simulink model "Modelo_benchmark"  (R2023a)
settings: Solver=VariableStepAuto  StartTime=0.0  StopTime=6250  RelTol=1e-3
values from neighbouring files (symbols this model uses):
  A = 0.0012    [control_temperatura.mat]    (also in var.m)
  C1_Q1 = 64.8931891795    [control_temperatura.mat]    (also in var.m = k3*Tau2)
  C1_Q2 = 0.0892445260493    [control_temperatura.mat]    (also in var.m = k1*k6)
  C2_Q1 = 0.558623321055    [control_temperatura.mat]    (also in var.m = k3)
  C_ff = GQ2T1cr/GQ1T1cr    [var.m]
  cp = 500    [control_temperatura.mat]    (also in var.m)
  e = zeros(1,iteraciones+ini)    [Codigo_discreto_ap.m]    (also in control_temperatura.mat = 0.9; var.m = 0.9)
  GQ1T1cr = tf(kcr1, [Taucr1 1])    [var.m]
  Hf1 = 0.01    [control_temperatura.mat]    (also in var.m)
  Hf2 = 0.004    [control_temperatura.mat]    (also in var.m)
  K_ap = 7.31538861094    [control_temperatura.mat]    (also in var.m = (2*delta*Taucr1*wn-1)/kcr1)
  K_cp = 1.15885597738    [control_temperatura.mat]    (also in var.m)
  m = 0.004    [control_temperatura.mat]    (also in var.m)
  P1_Q1 = 12978.6378359    [control_temperatura.mat]    (also in var.m = Tau1*Tau2)
  P1_Q2 = 12978.6378359    [control_temperatura.mat]    (also in var.m = Tau1*Tau2)
  P2_Q1 = 227.890937142    [control_temperatura.mat]    (also in var.m = Tau2+Tau1)
  P2_Q2 = 227.890937142    [control_temperatura.mat]    (also in var.m = Tau2+Tau1)
  P3_Q1 = 0.840856230771    [control_temperatura.mat]    (also in var.m = 1- k1*k4)
  P3_Q2 = 0.840856230771    [control_temperatura.mat]    (also in var.m = 1- k1*k4)
  T1i = 299.55    [control_temperatura.mat]    (also in var.m)
  T1o = 309.62355074    [control_temperatura.mat]    (also in var.m = x(1))
  T2i = 299.55    [control_temperatura.mat]    (also in var.m)
  TA = 299.55    [control_temperatura.mat]    (also in var.m)
  th = 5.67e-08    [control_temperatura.mat]    (also in var.m)
  Ti_ap = 23.6710802631    [control_temperatura.mat]    (also in var.m = (K_ap*kcr1)/(Taucr1*wn^2))
  Ti_cp = 165    [control_temperatura.mat]    (also in var.m)
  Tk = 273.15    [control_temperatura.mat]    (also in var.m)
  Tt_ap = 4.8652934406    [control_temperatura.mat]    (also in var.m = sqrt(Ti_ap))
  Tt_cp = 12.8452325787    [control_temperatura.mat]    (also in var.m = sqrt(Ti_cp))
  U = 1.4    [control_temperatura.mat]    (also in var.m)
undefined symbols (not defined in the file or in its folder): PID_Matlab
libraries: slpidlib x8, simulink_extras x6, simulink x4
(part 1 of 2)
settings Model: PacingRate=10  Creator=User  LastModifiedBy=User

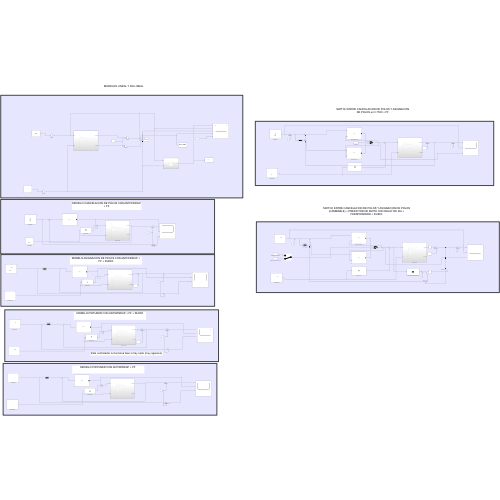
[thumbnail: Simulink's stored preview of the top-level diagram]
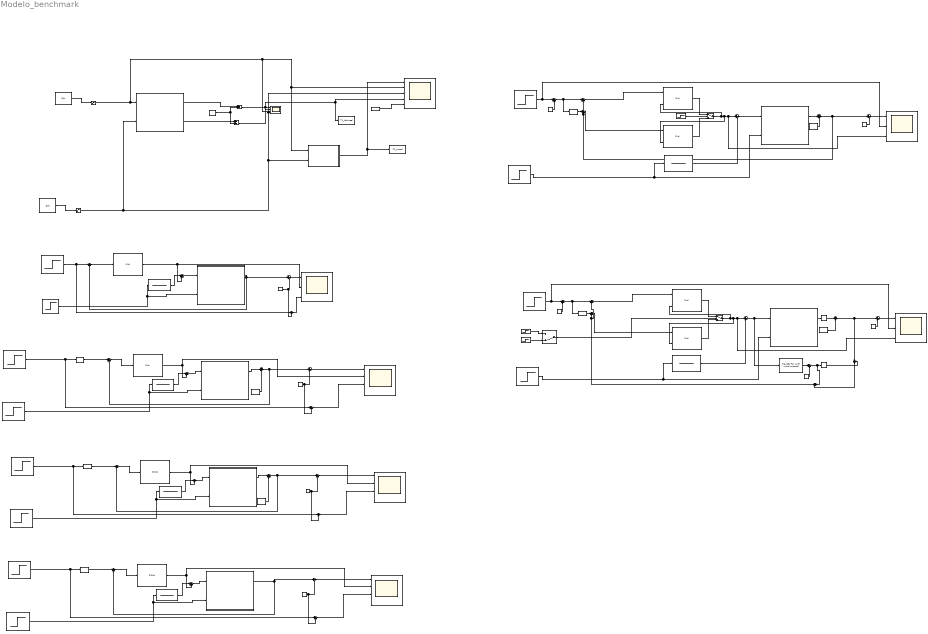
== system Modelo_benchmark ==
  note: SWITCH ENTRE CANCELACION DE POLOS Y ASIGNACION DE POLOS en t=1500 + FF
  note: MODELOS LINEAL Y NO LINEAL
  note: MODELO CANCELACION DE POLOS CON ANTIWINDUP + FF
  note: MODELO ASIGNACION DE POLOS CON ANTIWINDUP + FF + RUIDO
  note: SWITCH ENTRE CANCELACION DE POLOS Y ASIGNACION DE POLOS (CAMBIABLE) + PREDICTOR DE SMITH CON DELAY DE 40s + FEEDFORWARD + RUIDO
  note: MODELO PIDTUNER CON ANTIWINDUP + FF + RUIDO
  note: MODELO PIDTUNER CON ANTIWINDUP + FF
  note: Este controlador no funciona bien si hay ruido (muy agresivo)
  ASIGNACION POLOS : slpidlib/PID Controller  Controller=PI  Form=Parallel  TimeDomain=Continuous-time  UseExternalTs=off  SampleTime=-1  IntegratorMethod=Forward Euler  FilterMethod=Forward Euler  ControllerParametersSource=internal  P=K_ap  I=1/Ti_ap  UseKiTs=off  D=2  N=100  UseFilter=on  TunerSelectOption=Transfer Function Based (PID Tuner App)  InitialConditionSource=internal  InitialConditionForIntegrator=0  InitialConditionForFilter=0  DifferentiatorICPrevScaledInput=0  ExternalReset=none  TrackingMode=on  Kt=1/Tt_ap  LimitOutput=on  SatLimitsSource=internal  UpperSaturationLimit=100  LowerSaturationLimit=0  LinearizeAsGain=on  AntiWindupMode=back-calculation  Kb=1/Tt_ap  LimitIntegrator=off  UpperIntegratorSaturationLimit=inf  LowerIntegratorSaturationLimit=-inf  POutMin=[]  POutMax=[]  IOutMin=[]  IOutMax=[]  DOutMin=[]  DOutMax=[]  NOutMin=[]  NOutMax=[]  SumOutMin=[]  SumOutMax=[]  SaturationOutMin=[]  SaturationOutMax=[]  PParamMin=[]  PParamMax=[]  IParamMin=[]  IParamMax=[]  DParamMin=[]  DParamMax=[]  NParamMin=[]  NParamMax=[]  KbParamMin=[]  KbParamMax=[]  KtParamMin=[]  KtParamMax=[]  KbOutMin=[]  KbOutMax=[]  KtOutMin=[]  KtOutMax=[]  IntegratorOutMin=[]  IntegratorOutMax=[]  FilterOutMin=[]  FilterOutMax=[]  SumI1OutMin=[]  SumI1OutMax=[]  SumI2OutMin=[]  SumI2OutMax=[]  SumI3OutMin=[]  SumI3OutMax=[]  SumI4OutMin=[]  SumI4OutMax=[]  SumDOutMin=[]  SumDOutMax=[]  DifferentiatorOutMin=[]  DifferentiatorOutMax=[]  FilterDiffOutCoefMin=[]  FilterDiffOutCoefMax=[]  ReciprocalOutMin=[]  ReciprocalOutMax=[]  SumDenOutMin=[]  SumDenOutMax=[]  SumNumOutMin=[]  SumNumOutMax=[]  DivideOutMin=[]  DivideOutMax=[]  UdiffTsProdOutMin=[]  UdiffTsProdOutMax=[]  NTsProdOutMin=[]  NTsProdOutMax=[]  UintegralTsProdOutMin=[]  UintegralTsProdOutMax=[]  UngainTsProdOutMin=[]  UngainTsProdOutMax=[]  ClampingZeroOutDataTypeStr=Inherit: Inherit via back propagation  ClampingZeroOutMin=[]  ClampingZeroOutMax=[]  FilterDenConstantOutDataTypeStr=Inherit: Inherit via back propagation  FilterDenConstantOutMin=[]  FilterDenConstantOutMax=[]  PCopyOutDataTypeStr=Inherit: Inherit via back propagation  PCopyOutMin=[]  PCopyOutMax=[]  NCopyOutDataTypeStr=Inherit: Inherit via back propagation  NCopyOutMin=[]  NCopyOutMax=[]  IntegratorContinuousStateAttributes=''  IntegratorStateMustResolveToSignalObject=off  IntegratorRTWStateStorageClass=Auto  FilterContinuousStateAttributes=''  FilterStateMustResolveToSignalObject=off  FilterRTWStateStorageClass=Auto  ParallelPVariant=InternalParameters  IdealPVariant=Disabled  IVariant=InternalParameters  DVariant=Disabled  IntegratorVariant=Continuous  SatVariant=Enabled  AWVariant=BackCalculation  PCopyVariant=Disabled  TRVariant=Enabled  FdbkBlocksVariant=Forward  IdealPFdbkVariant=Disabled  SatFdbkVariant=Disabled  DerivativeFilterVariant=Disabled  NVariant=Disabled  NCopyVariant=Disabled_SignalSpec  FilterICVariant=Disabled  IntegratorICVariant=InternalICs  ExternalResetVariant=Disabled  TRSumVariant=TrackingMode  SumFdbkVariant=Disabled  SumVariant=Sum_PI  TsampFilterVariant=InternalTs  TsampNgainVariant=Passthrough  TsampIntegralVariant=Disabled_SignalSpec  ExternalSaturationOutDataTypeStr=Inherit: Same as second input
  ASIGNACION POLOS1 : slpidlib/PID Controller  Controller=PI  Form=Parallel  TimeDomain=Continuous-time  UseExternalTs=off  SampleTime=-1  IntegratorMethod=Forward Euler  FilterMethod=Forward Euler  ControllerParametersSource=internal  P=K_ap  I=1/Ti_ap  UseKiTs=off  D=2  N=100  UseFilter=on  TunerSelectOption=Transfer Function Based (PID Tuner App)  InitialConditionSource=internal  InitialConditionForIntegrator=0  InitialConditionForFilter=0  DifferentiatorICPrevScaledInput=0  ExternalReset=none  TrackingMode=on  Kt=1/Tt_ap  LimitOutput=on  SatLimitsSource=internal  UpperSaturationLimit=100  LowerSaturationLimit=0  LinearizeAsGain=on  AntiWindupMode=back-calculation  Kb=1/Tt_ap  LimitIntegrator=off  UpperIntegratorSaturationLimit=inf  LowerIntegratorSaturationLimit=-inf  POutMin=[]  POutMax=[]  IOutMin=[]  IOutMax=[]  DOutMin=[]  DOutMax=[]  NOutMin=[]  NOutMax=[]  SumOutMin=[]  SumOutMax=[]  SaturationOutMin=[]  SaturationOutMax=[]  PParamMin=[]  PParamMax=[]  IParamMin=[]  IParamMax=[]  DParamMin=[]  DParamMax=[]  NParamMin=[]  NParamMax=[]  KbParamMin=[]  KbParamMax=[]  KtParamMin=[]  KtParamMax=[]  KbOutMin=[]  KbOutMax=[]  KtOutMin=[]  KtOutMax=[]  IntegratorOutMin=[]  IntegratorOutMax=[]  FilterOutMin=[]  FilterOutMax=[]  SumI1OutMin=[]  SumI1OutMax=[]  SumI2OutMin=[]  SumI2OutMax=[]  SumI3OutMin=[]  SumI3OutMax=[]  SumI4OutMin=[]  SumI4OutMax=[]  SumDOutMin=[]  SumDOutMax=[]  DifferentiatorOutMin=[]  DifferentiatorOutMax=[]  FilterDiffOutCoefMin=[]  FilterDiffOutCoefMax=[]  ReciprocalOutMin=[]  ReciprocalOutMax=[]  SumDenOutMin=[]  SumDenOutMax=[]  SumNumOutMin=[]  SumNumOutMax=[]  DivideOutMin=[]  DivideOutMax=[]  UdiffTsProdOutMin=[]  UdiffTsProdOutMax=[]  NTsProdOutMin=[]  NTsProdOutMax=[]  UintegralTsProdOutMin=[]  UintegralTsProdOutMax=[]  UngainTsProdOutMin=[]  UngainTsProdOutMax=[]  ClampingZeroOutDataTypeStr=Inherit: Inherit via back propagation  ClampingZeroOutMin=[]  ClampingZeroOutMax=[]  FilterDenConstantOutDataTypeStr=Inherit: Inherit via back propagation  FilterDenConstantOutMin=[]  FilterDenConstantOutMax=[]  PCopyOutDataTypeStr=Inherit: Inherit via back propagation  PCopyOutMin=[]  PCopyOutMax=[]  NCopyOutDataTypeStr=Inherit: Inherit via back propagation  NCopyOutMin=[]  NCopyOutMax=[]  IntegratorContinuousStateAttributes=''  IntegratorStateMustResolveToSignalObject=off  IntegratorRTWStateStorageClass=Auto  FilterContinuousStateAttributes=''  FilterStateMustResolveToSignalObject=off  FilterRTWStateStorageClass=Auto  ParallelPVariant=InternalParameters  IdealPVariant=Disabled  IVariant=InternalParameters  DVariant=Disabled  IntegratorVariant=Continuous  SatVariant=Enabled  AWVariant=BackCalculation  PCopyVariant=Disabled  TRVariant=Enabled  FdbkBlocksVariant=Forward  IdealPFdbkVariant=Disabled  SatFdbkVariant=Disabled  DerivativeFilterVariant=Disabled  NVariant=Disabled  NCopyVariant=Disabled_SignalSpec  FilterICVariant=Disabled  IntegratorICVariant=InternalICs  ExternalResetVariant=Disabled  TRSumVariant=TrackingMode  SumFdbkVariant=Disabled  SumVariant=Sum_PI  TsampFilterVariant=InternalTs  TsampNgainVariant=Passthrough  TsampIntegralVariant=Disabled_SignalSpec  ExternalSaturationOutDataTypeStr=Inherit: Same as second input
  Band-Limited White Noise : simulink/Sources/Band-Limited White Noise  Cov=[0.2]  Ts=15  seed=[23341]
  Band-Limited White Noise1 : simulink/Sources/Band-Limited White Noise  Cov=[0.2]  Ts=10  seed=[23341]
  Band-Limited White Noise2 : simulink/Sources/Band-Limited White Noise  Cov=[0.2]  Ts=10  seed=[23341]
  Band-Limited White Noise3 : simulink/Sources/Band-Limited White Noise  Cov=[0.2]  Ts=15  seed=[23341]
  CANCELACION POLOS : slpidlib/PID Controller  Controller=PI  Form=Parallel  TimeDomain=Continuous-time  UseExternalTs=off  SampleTime=-1  IntegratorMethod=Forward Euler  FilterMethod=Forward Euler  ControllerParametersSource=internal  P=K_cp  I=1/Ti_cp  UseKiTs=off  D=2  N=100  UseFilter=on  TunerSelectOption=Transfer Function Based (PID Tuner App)  InitialConditionSource=internal  InitialConditionForIntegrator=0  InitialConditionForFilter=0  DifferentiatorICPrevScaledInput=0  ExternalReset=none  TrackingMode=on  Kt=1/Tt_cp  LimitOutput=on  SatLimitsSource=internal  UpperSaturationLimit=100  LowerSaturationLimit=0  LinearizeAsGain=on  AntiWindupMode=back-calculation  Kb=1/Tt_cp  LimitIntegrator=off  UpperIntegratorSaturationLimit=inf  LowerIntegratorSaturationLimit=-inf  POutMin=[]  POutMax=[]  IOutMin=[]  IOutMax=[]  DOutMin=[]  DOutMax=[]  NOutMin=[]  NOutMax=[]  SumOutMin=[]  SumOutMax=[]  SaturationOutMin=[]  SaturationOutMax=[]  PParamMin=[]  PParamMax=[]  IParamMin=[]  IParamMax=[]  DParamMin=[]  DParamMax=[]  NParamMin=[]  NParamMax=[]  KbParamMin=[]  KbParamMax=[]  KtParamMin=[]  KtParamMax=[]  KbOutMin=[]  KbOutMax=[]  KtOutMin=[]  KtOutMax=[]  IntegratorOutMin=[]  IntegratorOutMax=[]  FilterOutMin=[]  FilterOutMax=[]  SumI1OutMin=[]  SumI1OutMax=[]  SumI2OutMin=[]  SumI2OutMax=[]  SumI3OutMin=[]  SumI3OutMax=[]  SumI4OutMin=[]  SumI4OutMax=[]  SumDOutMin=[]  SumDOutMax=[]  DifferentiatorOutMin=[]  DifferentiatorOutMax=[]  FilterDiffOutCoefMin=[]  FilterDiffOutCoefMax=[]  ReciprocalOutMin=[]  ReciprocalOutMax=[]  SumDenOutMin=[]  SumDenOutMax=[]  SumNumOutMin=[]  SumNumOutMax=[]  DivideOutMin=[]  DivideOutMax=[]  UdiffTsProdOutMin=[]  UdiffTsProdOutMax=[]  NTsProdOutMin=[]  NTsProdOutMax=[]  UintegralTsProdOutMin=[]  UintegralTsProdOutMax=[]  UngainTsProdOutMin=[]  UngainTsProdOutMax=[]  ClampingZeroOutDataTypeStr=Inherit: Inherit via back propagation  ClampingZeroOutMin=[]  ClampingZeroOutMax=[]  FilterDenConstantOutDataTypeStr=Inherit: Inherit via back propagation  FilterDenConstantOutMin=[]  FilterDenConstantOutMax=[]  PCopyOutDataTypeStr=Inherit: Inherit via back propagation  PCopyOutMin=[]  PCopyOutMax=[]  NCopyOutDataTypeStr=Inherit: Inherit via back propagation  NCopyOutMin=[]  NCopyOutMax=[]  IntegratorContinuousStateAttributes=''  IntegratorStateMustResolveToSignalObject=off  IntegratorRTWStateStorageClass=Auto  FilterContinuousStateAttributes=''  FilterStateMustResolveToSignalObject=off  FilterRTWStateStorageClass=Auto  ParallelPVariant=InternalParameters  IdealPVariant=Disabled  IVariant=InternalParameters  DVariant=Disabled  IntegratorVariant=Continuous  SatVariant=Enabled  AWVariant=BackCalculation  PCopyVariant=Disabled  TRVariant=Enabled  FdbkBlocksVariant=Forward  IdealPFdbkVariant=Disabled  SatFdbkVariant=Disabled  DerivativeFilterVariant=Disabled  NVariant=Disabled  NCopyVariant=Disabled_SignalSpec  FilterICVariant=Disabled  IntegratorICVariant=InternalICs  ExternalResetVariant=Disabled  TRSumVariant=TrackingMode  SumFdbkVariant=Disabled  SumVariant=Sum_PI  TsampFilterVariant=InternalTs  TsampNgainVariant=Passthrough  TsampIntegralVariant=Disabled_SignalSpec  ExternalSaturationOutDataTypeStr=Inherit: Same as second input
  CANCELACION POLOS1 : slpidlib/PID Controller  Controller=PI  Form=Parallel  TimeDomain=Continuous-time  UseExternalTs=off  SampleTime=-1  IntegratorMethod=Forward Euler  FilterMethod=Forward Euler  ControllerParametersSource=internal  P=K_cp  I=1/Ti_cp  UseKiTs=off  D=2  N=100  UseFilter=on  TunerSelectOption=Transfer Function Based (PID Tuner App)  InitialConditionSource=internal  InitialConditionForIntegrator=0  InitialConditionForFilter=0  DifferentiatorICPrevScaledInput=0  ExternalReset=none  TrackingMode=on  Kt=1/Tt_cp  LimitOutput=on  SatLimitsSource=internal  UpperSaturationLimit=100  LowerSaturationLimit=0  LinearizeAsGain=on  AntiWindupMode=back-calculation  Kb=1/Tt_cp  LimitIntegrator=off  UpperIntegratorSaturationLimit=inf  LowerIntegratorSaturationLimit=-inf  POutMin=[]  POutMax=[]  IOutMin=[]  IOutMax=[]  DOutMin=[]  DOutMax=[]  NOutMin=[]  NOutMax=[]  SumOutMin=[]  SumOutMax=[]  SaturationOutMin=[]  SaturationOutMax=[]  PParamMin=[]  PParamMax=[]  IParamMin=[]  IParamMax=[]  DParamMin=[]  DParamMax=[]  NParamMin=[]  NParamMax=[]  KbParamMin=[]  KbParamMax=[]  KtParamMin=[]  KtParamMax=[]  KbOutMin=[]  KbOutMax=[]  KtOutMin=[]  KtOutMax=[]  IntegratorOutMin=[]  IntegratorOutMax=[]  FilterOutMin=[]  FilterOutMax=[]  SumI1OutMin=[]  SumI1OutMax=[]  SumI2OutMin=[]  SumI2OutMax=[]  SumI3OutMin=[]  SumI3OutMax=[]  SumI4OutMin=[]  SumI4OutMax=[]  SumDOutMin=[]  SumDOutMax=[]  DifferentiatorOutMin=[]  DifferentiatorOutMax=[]  FilterDiffOutCoefMin=[]  FilterDiffOutCoefMax=[]  ReciprocalOutMin=[]  ReciprocalOutMax=[]  SumDenOutMin=[]  SumDenOutMax=[]  SumNumOutMin=[]  SumNumOutMax=[]  DivideOutMin=[]  DivideOutMax=[]  UdiffTsProdOutMin=[]  UdiffTsProdOutMax=[]  NTsProdOutMin=[]  NTsProdOutMax=[]  UintegralTsProdOutMin=[]  UintegralTsProdOutMax=[]  UngainTsProdOutMin=[]  UngainTsProdOutMax=[]  ClampingZeroOutDataTypeStr=Inherit: Inherit via back propagation  ClampingZeroOutMin=[]  ClampingZeroOutMax=[]  FilterDenConstantOutDataTypeStr=Inherit: Inherit via back propagation  FilterDenConstantOutMin=[]  FilterDenConstantOutMax=[]  PCopyOutDataTypeStr=Inherit: Inherit via back propagation  PCopyOutMin=[]  PCopyOutMax=[]  NCopyOutDataTypeStr=Inherit: Inherit via back propagation  NCopyOutMin=[]  NCopyOutMax=[]  IntegratorContinuousStateAttributes=''  IntegratorStateMustResolveToSignalObject=off  IntegratorRTWStateStorageClass=Auto  FilterContinuousStateAttributes=''  FilterStateMustResolveToSignalObject=off  FilterRTWStateStorageClass=Auto  ParallelPVariant=InternalParameters  IdealPVariant=Disabled  IVariant=InternalParameters  DVariant=Disabled  IntegratorVariant=Continuous  SatVariant=Enabled  AWVariant=BackCalculation  PCopyVariant=Disabled  TRVariant=Enabled  FdbkBlocksVariant=Forward  IdealPFdbkVariant=Disabled  SatFdbkVariant=Disabled  DerivativeFilterVariant=Disabled  NVariant=Disabled  NCopyVariant=Disabled_SignalSpec  FilterICVariant=Disabled  IntegratorICVariant=InternalICs  ExternalResetVariant=Disabled  TRSumVariant=TrackingMode  SumFdbkVariant=Disabled  SumVariant=Sum_PI  TsampFilterVariant=InternalTs  TsampNgainVariant=Passthrough  TsampIntegralVariant=Disabled_SignalSpec  ExternalSaturationOutDataTypeStr=Inherit: Same as second input
  Constant{1..6,8..9,14} (9 alike) : Constant  Value=Tk
  Constant7 : Constant  Value=T1i
  Controlador FF{,1..5} (6 alike) : TransferFcn  Numerator=C_ff.Numerator{:}  Denominator=C_ff.Denominator{:}
  From Workspace : FromWorkspace  VariableName=Q1t  SampleTime=0.5
  From Workspace1 : FromWorkspace  VariableName=Q2t  SampleTime=0.5
  From Workspace2 : FromWorkspace  VariableName=T1t
  "MODELO SISTEMA CURVA REACCION " : simulink_extras/Additional Linear/Transfer Fcn (with initial outputs)  N=GQ1T1cr.Numerator{:}  D=GQ1T1cr.Denominator{:}  Y0=0  U0=0
  Manual Switch : ManualSwitch  CurrentSetting=0
  Modelo_ Nolineal : Subsystem
  Modelo_ Nolineal1 : Subsystem
  Modelo_ Nolineal2 : Subsystem
  Modelo_ Nolineal3 : Subsystem
  Modelo_ Nolineal4 : Subsystem
  Modelo_ Nolineal5 : Subsystem
  Modelo_ Nolineal6 : Subsystem
  PERTURBACION : Step  Time=4500  After=15  SampleTime=0
  PERTURBACION{1..5} (5 alike) : Step  Time=4500  After=100  SampleTime=0
  PID Controller : slpidlib/PID Controller  Controller=PI  Form=Parallel  TimeDomain=Continuous-time  UseExternalTs=off  SampleTime=-1  IntegratorMethod=Forward Euler  FilterMethod=Forward Euler  ControllerParametersSource=internal  P=K_cp  I=1/Ti_cp  UseKiTs=off  D=2  N=100  UseFilter=on  TunerSelectOption=Transfer Function Based (PID Tuner App)  InitialConditionSource=internal  InitialConditionForIntegrator=0  InitialConditionForFilter=0  DifferentiatorICPrevScaledInput=0  ExternalReset=none  TrackingMode=off  Kt=1  LimitOutput=on  SatLimitsSource=internal  UpperSaturationLimit=100  LowerSaturationLimit=0  LinearizeAsGain=on  AntiWindupMode=back-calculation  Kb=1/Tt_cp  LimitIntegrator=off  UpperIntegratorSaturationLimit=inf  LowerIntegratorSaturationLimit=-inf  POutMin=[]  POutMax=[]  IOutMin=[]  IOutMax=[]  DOutMin=[]  DOutMax=[]  NOutMin=[]  NOutMax=[]  SumOutMin=[]  SumOutMax=[]  SaturationOutMin=[]  SaturationOutMax=[]  PParamMin=[]  PParamMax=[]  IParamMin=[]  IParamMax=[]  DParamMin=[]  DParamMax=[]  NParamMin=[]  NParamMax=[]  KbParamMin=[]  KbParamMax=[]  KtParamMin=[]  KtParamMax=[]  KbOutMin=[]  KbOutMax=[]  KtOutMin=[]  KtOutMax=[]  IntegratorOutMin=[]  IntegratorOutMax=[]  FilterOutMin=[]  FilterOutMax=[]  SumI1OutMin=[]  SumI1OutMax=[]  SumI2OutMin=[]  SumI2OutMax=[]  SumI3OutMin=[]  SumI3OutMax=[]  SumI4OutMin=[]  SumI4OutMax=[]  SumDOutMin=[]  SumDOutMax=[]  DifferentiatorOutMin=[]  DifferentiatorOutMax=[]  FilterDiffOutCoefMin=[]  FilterDiffOutCoefMax=[]  ReciprocalOutMin=[]  ReciprocalOutMax=[]  SumDenOutMin=[]  SumDenOutMax=[]  SumNumOutMin=[]  SumNumOutMax=[]  DivideOutMin=[]  DivideOutMax=[]  UdiffTsProdOutMin=[]  UdiffTsProdOutMax=[]  NTsProdOutMin=[]  NTsProdOutMax=[]  UintegralTsProdOutMin=[]  UintegralTsProdOutMax=[]  UngainTsProdOutMin=[]  UngainTsProdOutMax=[]  ClampingZeroOutDataTypeStr=Inherit: Inherit via back propagation  ClampingZeroOutMin=[]  ClampingZeroOutMax=[]  FilterDenConstantOutDataTypeStr=Inherit: Inherit via back propagation  FilterDenConstantOutMin=[]  FilterDenConstantOutMax=[]  PCopyOutDataTypeStr=Inherit: Inherit via back propagation  PCopyOutMin=[]  PCopyOutMax=[]  NCopyOutDataTypeStr=Inherit: Inherit via back propagation  NCopyOutMin=[]  NCopyOutMax=[]  IntegratorContinuousStateAttributes=''  IntegratorStateMustResolveToSignalObject=off  IntegratorRTWStateStorageClass=Auto  FilterContinuousStateAttributes=''  FilterStateMustResolveToSignalObject=off  FilterRTWStateStorageClass=Auto  ParallelPVariant=InternalParameters  IdealPVariant=Disabled  IVariant=InternalParameters  DVariant=Disabled  IntegratorVariant=Continuous  SatVariant=Enabled  AWVariant=BackCalculation  PCopyVariant=Disabled  TRVariant=Disabled  FdbkBlocksVariant=Forward  IdealPFdbkVariant=Disabled  SatFdbkVariant=Disabled  DerivativeFilterVariant=Disabled  NVariant=Disabled  NCopyVariant=Disabled_SignalSpec  FilterICVariant=Disabled  IntegratorICVariant=InternalICs  ExternalResetVariant=Disabled  TRSumVariant=Passthrough  SumFdbkVariant=Disabled  SumVariant=Sum_PI  TsampFilterVariant=InternalTs  TsampNgainVariant=Passthrough  TsampIntegralVariant=Disabled_SignalSpec  ExternalSaturationOutDataTypeStr=Inherit: Same as second input
  PID Controller1 : slpidlib/PID Controller  Controller=PI  Form=Parallel  TimeDomain=Continuous-time  UseExternalTs=off  SampleTime=-1  IntegratorMethod=Forward Euler  FilterMethod=Forward Euler  ControllerParametersSource=internal  P=K_ap  I=1/Ti_ap  UseKiTs=off  D=2  N=100  UseFilter=on  TunerSelectOption=Transfer Function Based (PID Tuner App)  InitialConditionSource=internal  InitialConditionForIntegrator=0  InitialConditionForFilter=0  DifferentiatorICPrevScaledInput=0  ExternalReset=none  TrackingMode=off  Kt=1  LimitOutput=on  SatLimitsSource=internal  UpperSaturationLimit=100  LowerSaturationLimit=0  LinearizeAsGain=on  AntiWindupMode=back-calculation  Kb=1/Tt_ap  LimitIntegrator=off  UpperIntegratorSaturationLimit=inf  LowerIntegratorSaturationLimit=-inf  POutMin=[]  POutMax=[]  IOutMin=[]  IOutMax=[]  DOutMin=[]  DOutMax=[]  NOutMin=[]  NOutMax=[]  SumOutMin=[]  SumOutMax=[]  SaturationOutMin=[]  SaturationOutMax=[]  PParamMin=[]  PParamMax=[]  IParamMin=[]  IParamMax=[]  DParamMin=[]  DParamMax=[]  NParamMin=[]  NParamMax=[]  KbParamMin=[]  KbParamMax=[]  KtParamMin=[]  KtParamMax=[]  KbOutMin=[]  KbOutMax=[]  KtOutMin=[]  KtOutMax=[]  IntegratorOutMin=[]  IntegratorOutMax=[]  FilterOutMin=[]  FilterOutMax=[]  SumI1OutMin=[]  SumI1OutMax=[]  SumI2OutMin=[]  SumI2OutMax=[]  SumI3OutMin=[]  SumI3OutMax=[]  SumI4OutMin=[]  SumI4OutMax=[]  SumDOutMin=[]  SumDOutMax=[]  DifferentiatorOutMin=[]  DifferentiatorOutMax=[]  FilterDiffOutCoefMin=[]  FilterDiffOutCoefMax=[]  ReciprocalOutMin=[]  ReciprocalOutMax=[]  SumDenOutMin=[]  SumDenOutMax=[]  SumNumOutMin=[]  SumNumOutMax=[]  DivideOutMin=[]  DivideOutMax=[]  UdiffTsProdOutMin=[]  UdiffTsProdOutMax=[]  NTsProdOutMin=[]  NTsProdOutMax=[]  UintegralTsProdOutMin=[]  UintegralTsProdOutMax=[]  UngainTsProdOutMin=[]  UngainTsProdOutMax=[]  ClampingZeroOutDataTypeStr=Inherit: Inherit via back propagation  ClampingZeroOutMin=[]  ClampingZeroOutMax=[]  FilterDenConstantOutDataTypeStr=Inherit: Inherit via back propagation  FilterDenConstantOutMin=[]  FilterDenConstantOutMax=[]  PCopyOutDataTypeStr=Inherit: Inherit via back propagation  PCopyOutMin=[]  PCopyOutMax=[]  NCopyOutDataTypeStr=Inherit: Inherit via back propagation  NCopyOutMin=[]  NCopyOutMax=[]  IntegratorContinuousStateAttributes=''  IntegratorStateMustResolveToSignalObject=off  IntegratorRTWStateStorageClass=Auto  FilterContinuousStateAttributes=''  FilterStateMustResolveToSignalObject=off  FilterRTWStateStorageClass=Auto  ParallelPVariant=InternalParameters  IdealPVariant=Disabled  IVariant=InternalParameters  DVariant=Disabled  IntegratorVariant=Continuous  SatVariant=Enabled  AWVariant=BackCalculation  PCopyVariant=Disabled  TRVariant=Disabled  FdbkBlocksVariant=Forward  IdealPFdbkVariant=Disabled  SatFdbkVariant=Disabled  DerivativeFilterVariant=Disabled  NVariant=Disabled  NCopyVariant=Disabled_SignalSpec  FilterICVariant=Disabled  IntegratorICVariant=InternalICs  ExternalResetVariant=Disabled  TRSumVariant=Passthrough  SumFdbkVariant=Disabled  SumVariant=Sum_PI  TsampFilterVariant=InternalTs  TsampNgainVariant=Passthrough  TsampIntegralVariant=Disabled_SignalSpec  ExternalSaturationOutDataTypeStr=Inherit: Same as second input
  PID Controller2 : slpidlib/PID Controller  Controller=PID  Form=Parallel  TimeDomain=Continuous-time  UseExternalTs=off  SampleTime=-1  IntegratorMethod=Forward Euler  FilterMethod=Forward Euler  ControllerParametersSource=internal  P=PID_Matlab.Kp  I=PID_Matlab.Ki  UseKiTs=off  D=PID_Matlab.Kd  N=PID_Matlab.Tf  UseFilter=on  TunerSelectOption=Transfer Function Based (PID Tuner App)  InitialConditionSource=internal  InitialConditionForIntegrator=0  InitialConditionForFilter=0  DifferentiatorICPrevScaledInput=0  ExternalReset=none  TrackingMode=off  Kt=1  LimitOutput=on  SatLimitsSource=internal  UpperSaturationLimit=100  LowerSaturationLimit=0  LinearizeAsGain=on  AntiWindupMode=back-calculation  Kb=1/Tt_ap  LimitIntegrator=off  UpperIntegratorSaturationLimit=inf  LowerIntegratorSaturationLimit=-inf  POutMin=[]  POutMax=[]  IOutMin=[]  IOutMax=[]  DOutMin=[]  DOutMax=[]  NOutMin=[]  NOutMax=[]  SumOutMin=[]  SumOutMax=[]  SaturationOutMin=[]  SaturationOutMax=[]  PParamMin=[]  PParamMax=[]  IParamMin=[]  IParamMax=[]  DParamMin=[]  DParamMax=[]  NParamMin=[]  NParamMax=[]  KbParamMin=[]  KbParamMax=[]  KtParamMin=[]  KtParamMax=[]  KbOutMin=[]  KbOutMax=[]  KtOutMin=[]  KtOutMax=[]  IntegratorOutMin=[]  IntegratorOutMax=[]  FilterOutMin=[]  FilterOutMax=[]  SumI1OutMin=[]  SumI1OutMax=[]  SumI2OutMin=[]  SumI2OutMax=[]  SumI3OutMin=[]  SumI3OutMax=[]  SumI4OutMin=[]  SumI4OutMax=[]  SumDOutMin=[]  SumDOutMax=[]  DifferentiatorOutMin=[]  DifferentiatorOutMax=[]  FilterDiffOutCoefMin=[]  FilterDiffOutCoefMax=[]  ReciprocalOutMin=[]  ReciprocalOutMax=[]  SumDenOutMin=[]  SumDenOutMax=[]  SumNumOutMin=[]  SumNumOutMax=[]  DivideOutMin=[]  DivideOutMax=[]  UdiffTsProdOutMin=[]  UdiffTsProdOutMax=[]  NTsProdOutMin=[]  NTsProdOutMax=[]  UintegralTsProdOutMin=[]  UintegralTsProdOutMax=[]  UngainTsProdOutMin=[]  UngainTsProdOutMax=[]  ClampingZeroOutDataTypeStr=Inherit: Inherit via back propagation  ClampingZeroOutMin=[]  ClampingZeroOutMax=[]  FilterDenConstantOutDataTypeStr=Inherit: Inherit via back propagation  FilterDenConstantOutMin=[]  FilterDenConstantOutMax=[]  PCopyOutDataTypeStr=Inherit: Inherit via back propagation  PCopyOutMin=[]  PCopyOutMax=[]  NCopyOutDataTypeStr=Inherit: Inherit via back propagation  NCopyOutMin=[]  NCopyOutMax=[]  IntegratorContinuousStateAttributes=''  IntegratorStateMustResolveToSignalObject=off  IntegratorRTWStateStorageClass=Auto  FilterContinuousStateAttributes=''  FilterStateMustResolveToSignalObject=off  FilterRTWStateStorageClass=Auto  ParallelPVariant=InternalParameters  IdealPVariant=Disabled  IVariant=InternalParameters  DVariant=InternalParameters  IntegratorVariant=Continuous  SatVariant=Enabled  AWVariant=BackCalculation  PCopyVariant=Disabled  TRVariant=Disabled  FdbkBlocksVariant=Forward  IdealPFdbkVariant=Disabled  SatFdbkVariant=Disabled  DerivativeFilterVariant=ContFilter  NVariant=InternalParameters  NCopyVariant=Disabled  FilterICVariant=InternalICsFilter  IntegratorICVariant=InternalICs  ExternalResetVariant=Disabled  TRSumVariant=Passthrough  SumFdbkVariant=Disabled  SumVariant=Sum_PID  TsampFilterVariant=InternalTs  TsampNgainVariant=Passthrough  TsampIntegralVariant=Disabled_SignalSpec  ExternalSaturationOutDataTypeStr=Inherit: Same as second input
  PID Controller3 : slpidlib/PID Controller  Controller=PID  Form=Parallel  TimeDomain=Continuous-time  UseExternalTs=off  SampleTime=-1  IntegratorMethod=Forward Euler  FilterMethod=Forward Euler  ControllerParametersSource=internal  P=PID_Matlab.Kp  I=PID_Matlab.Ki  UseKiTs=off  D=PID_Matlab.Kd  N=PID_Matlab.Tf  UseFilter=on  TunerSelectOption=Transfer Function Based (PID Tuner App)  InitialConditionSource=internal  InitialConditionForIntegrator=0  InitialConditionForFilter=0  DifferentiatorICPrevScaledInput=0  ExternalReset=none  TrackingMode=off  Kt=1  LimitOutput=on  SatLimitsSource=internal  UpperSaturationLimit=100  LowerSaturationLimit=0  LinearizeAsGain=on  AntiWindupMode=back-calculation  Kb=1/Tt_ap  LimitIntegrator=off  UpperIntegratorSaturationLimit=inf  LowerIntegratorSaturationLimit=-inf  POutMin=[]  POutMax=[]  IOutMin=[]  IOutMax=[]  DOutMin=[]  DOutMax=[]  NOutMin=[]  NOutMax=[]  SumOutMin=[]  SumOutMax=[]  SaturationOutMin=[]  SaturationOutMax=[]  PParamMin=[]  PParamMax=[]  IParamMin=[]  IParamMax=[]  DParamMin=[]  DParamMax=[]  NParamMin=[]  NParamMax=[]  KbParamMin=[]  KbParamMax=[]  KtParamMin=[]  KtParamMax=[]  KbOutMin=[]  KbOutMax=[]  KtOutMin=[]  KtOutMax=[]  IntegratorOutMin=[]  IntegratorOutMax=[]  FilterOutMin=[]  FilterOutMax=[]  SumI1OutMin=[]  SumI1OutMax=[]  SumI2OutMin=[]  SumI2OutMax=[]  SumI3OutMin=[]  SumI3OutMax=[]  SumI4OutMin=[]  SumI4OutMax=[]  SumDOutMin=[]  SumDOutMax=[]  DifferentiatorOutMin=[]  DifferentiatorOutMax=[]  FilterDiffOutCoefMin=[]  FilterDiffOutCoefMax=[]  ReciprocalOutMin=[]  ReciprocalOutMax=[]  SumDenOutMin=[]  SumDenOutMax=[]  SumNumOutMin=[]  SumNumOutMax=[]  DivideOutMin=[]  DivideOutMax=[]  UdiffTsProdOutMin=[]  UdiffTsProdOutMax=[]  NTsProdOutMin=[]  NTsProdOutMax=[]  UintegralTsProdOutMin=[]  UintegralTsProdOutMax=[]  UngainTsProdOutMin=[]  UngainTsProdOutMax=[]  ClampingZeroOutDataTypeStr=Inherit: Inherit via back propagation  ClampingZeroOutMin=[]  ClampingZeroOutMax=[]  FilterDenConstantOutDataTypeStr=Inherit: Inherit via back propagation  FilterDenConstantOutMin=[]  FilterDenConstantOutMax=[]  PCopyOutDataTypeStr=Inherit: Inherit via back propagation  PCopyOutMin=[]  PCopyOutMax=[]  NCopyOutDataTypeStr=Inherit: Inherit via back propagation  NCopyOutMin=[]  NCopyOutMax=[]  IntegratorContinuousStateAttributes=''  IntegratorStateMustResolveToSignalObject=off  IntegratorRTWStateStorageClass=Auto  FilterContinuousStateAttributes=''  FilterStateMustResolveToSignalObject=off  FilterRTWStateStorageClass=Auto  ParallelPVariant=InternalParameters  IdealPVariant=Disabled  IVariant=InternalParameters  DVariant=InternalParameters  IntegratorVariant=Continuous  SatVariant=Enabled  AWVariant=BackCalculation  PCopyVariant=Disabled  TRVariant=Disabled  FdbkBlocksVariant=Forward  IdealPFdbkVariant=Disabled  SatFdbkVariant=Disabled  DerivativeFilterVariant=ContFilter  NVariant=InternalParameters  NCopyVariant=Disabled  FilterICVariant=InternalICsFilter  IntegratorICVariant=InternalICs  ExternalResetVariant=Disabled  TRSumVariant=Passthrough  SumFdbkVariant=Disabled  SumVariant=Sum_PID  TsampFilterVariant=InternalTs  TsampNgainVariant=Passthrough  TsampIntegralVariant=Disabled_SignalSpec  ExternalSaturationOutDataTypeStr=Inherit: Same as second input
  PRIMERO ASIGNACION POLOS : Step  Time=1500  SampleTime=0
  PRIMERO CANCELACION POLOS : Step  Time=1500  Before=1  After=0  SampleTime=0
  Q1_Modelo : Saturate  UpperLimit=100  LowerLimit=0
  Q2_Modelo : Saturate  UpperLimit=100  LowerLimit=0
  REFERENCIA : Step  Time=2000  Before=50+ Tk  After=80+ Tk  SampleTime=0
  REFERENCIA (Cº){,1..3} (4 alike) : Sum  Inputs=|+-
  REFERENCIA1 : Step  Time=2000  Before=40+ Tk  After=85+ Tk  SampleTime=0
  REFERENCIA2 : Step  Time=2000  Before=40  After=85  SampleTime=0
  REFERENCIA3 : Step  Time=1500  SampleTime=0
  REFERENCIA4 : Step  Time=2000  Before=30  After=50  SampleTime=0
  REFERENCIA5 : Step  Time=2000  Before=40+ Tk  After=85+ Tk  SampleTime=0
  REFERENCIA6 : Step  Time=2000  Before=40+ Tk  After=85+ Tk  SampleTime=0
  SALIDA (Cº){,1,3,6,9,12,14} (7 alike) : Sum  Inputs=|+-
  SALIDA (Cº){2,4..5,7..8,10..11,13} (8 alike) : Sum  Inputs=|++
  Scope{,3,6..7} (4 alike) : Scope  NumInputPorts=4
  Scope1 : Scope  NumInputPorts=5
  Scope2 : Scope  NumInputPorts=3
  Scope4 : Scope  NumInputPorts=3
  Scope5 : Scope  NumInputPorts=3
  Subsystem : Subsystem
  Sum{,1,4..10,12} (10 alike) : Sum  Inputs=|+-
  Sum{2..3,11,13} (4 alike) : Sum  Inputs=|-+
  Switch : Switch  Criteria=u2 > Threshold  SaturateOnIntegerOverflow=off  InputSameDT=off
  Switch1 : Switch  Criteria=u2 > Threshold  SaturateOnIntegerOverflow=off  InputSameDT=off
  T1_nolineal : Sum  Inputs=+-
  T2_nolineal : Sum  Inputs=+-
  To Workspace : ToWorkspace  VariableName=T1_Lineal  SaveFormat=Timeseries  SampleTime=-1
  To Workspace3 : ToWorkspace  VariableName=T1_NoLineal  SaveFormat=Timeseries  SampleTime=-1
  Transfer Fcn (with initial outputs){,1,3..4} (4 alike) : simulink_extras/Additional Linear/Transfer Fcn (with initial outputs)  N=[1]  D="[Ti_ap  1]"  Y0=40+ Tk  U0=0
  Transfer Fcn (with initial outputs)2 : simulink_extras/Additional Linear/Transfer Fcn (with initial outputs)  N=[1]  D="[Ti_ap  1]"  Y0=30+Tk  U0=0
  Transport Delay : TransportDelay  DelayTime=40  InitialOutput=T1i
  Transport Delay1 : TransportDelay  DelayTime=40  InitialOutput=T1i
  wires:
  Q2_Modelo/1 -> Modelo_ Nolineal/2(Q2), Scope1/3, Scope/4, Subsystem/2(Q2)
  T1_nolineal/1 -> Scope1/4, To Workspace3/1, Scope/1
  Constant14/1 -> T1_nolineal/2, T2_nolineal/2
  Q1_Modelo/1 -> Scope/3, Subsystem/1(Q1), Scope1/2, Modelo_ Nolineal/1(Q1)
  From Workspace1/1 -> Q2_Modelo/1
  T2_nolineal/1 -> Scope/2
  From Workspace/1 -> Q1_Modelo/1
  From Workspace2/1 -> Scope1/5
  Modelo_ Nolineal/1(T1_Nolineal) -> T1_nolineal/1
  Modelo_ Nolineal/2(T2_Nlineal) -> T2_nolineal/1
  Subsystem/1(T1_Lineal) -> To Workspace/1, Scope1/1
  Modelo_ Nolineal1/1(T1_Nolineal) -> SALIDA (Cº)/1, Sum/2
  Sum/1 -> PID Controller/1
  PERTURBACION/1 -> Controlador FF1/1, Modelo_ Nolineal1/2(Q2)
  SALIDA (Cº)/1 -> Scope2/1
  REFERENCIA/1 -> REFERENCIA (Cº)/1, Sum/1
  Constant2/1 -> SALIDA (Cº)/2, REFERENCIA (Cº)/2
  REFERENCIA (Cº)/1 -> Scope2/3
  PERTURBACION1/1 -> Controlador FF/1, Modelo_ Nolineal2/2(Q2)
  Constant1/1 -> SALIDA (Cº)1/2, REFERENCIA (Cº)1/2
  REFERENCIA1/1 -> Transfer Fcn (with initial outputs)/1, REFERENCIA (Cº)1/1
  REFERENCIA (Cº)1/1 -> Scope3/3
  SALIDA (Cº)1/1 -> Scope3/1
  PID Controller1/1 -> Scope3/2, Sum2/2
  Sum2/1 -> Modelo_ Nolineal2/1(Q1)
  Controlador FF1/1 -> Sum3/1
  PID Controller/1 -> Sum3/2, Scope2/2
  Sum3/1 -> Modelo_ Nolineal1/1(Q1)
  Sum1/1 -> PID Controller1/1
  Transfer Fcn (with initial outputs)/1 -> Sum1/1
  Controlador FF/1 -> Sum2/1
  Band-Limited White Noise/1 -> SALIDA (Cº)2/2
  SALIDA (Cº)2/1 -> Sum1/2, SALIDA (Cº)1/1
  Modelo_ Nolineal2/1(T1_Nolineal) -> SALIDA (Cº)2/1
  CANCELACION POLOS/1 -> Switch/1
  Switch/1 -> CANCELACION POLOS/2, Scope4/3, Sum6/1, ASIGNACION POLOS/2
  Modelo_ Nolineal3/1(T1_Nolineal) -> SALIDA (Cº)5/1
  Sum4/1 -> CANCELACION POLOS/1
  Sum5/1 -> ASIGNACION POLOS/1
  Transfer Fcn (with initial outputs)1/1 -> Sum5/1
  ASIGNACION POLOS/1 -> Switch/3
  REFERENCIA3/1 -> Switch/2
  Sum6/1 -> Modelo_ Nolineal3/1(Q1)
  Controlador FF2/1 -> Sum6/2
  PERTURBACION2/1 -> Controlador FF2/1, Modelo_ Nolineal3/2(Q2)
  Constant3/1 -> SALIDA (Cº)3/2
  SALIDA (Cº)3/1 -> Scope4/1
  Constant4/1 -> SALIDA (Cº)4/2
  REFERENCIA2/1 -> Scope4/2, SALIDA (Cº)4/1
  SALIDA (Cº)4/1 -> Transfer Fcn (with initial outputs)1/1, Sum4/1
  Band-Limited White Noise1/1 -> SALIDA (Cº)5/2
  SALIDA (Cº)5/1 -> SALIDA (Cº)3/1, Sum5/2, Sum4/2
  SALIDA (Cº)8/1 -> SALIDA (Cº)6/1, SALIDA (Cº)9/1
  SALIDA (Cº)7/1 -> Transfer Fcn (with initial outputs)2/1, Sum7/1
  CANCELACION POLOS1/1 -> Switch1/1
  Constant5/1 -> SALIDA (Cº)6/2
  Constant6/1 -> SALIDA (Cº)7/2
  Switch1/1 -> CANCELACION POLOS1/2, Scope5/3, Sum9/1, ASIGNACION POLOS1/2
  PERTURBACION3/1 -> Controlador FF3/1, Modelo_ Nolineal4/2(Q2)
  REFERENCIA4/1 -> Scope5/2, SALIDA (Cº)7/1
  Transfer Fcn (with initial outputs)2/1 -> Sum8/1
  Band-Limited White Noise2/1 -> SALIDA (Cº)8/2
  Modelo_ Nolineal4/1(T1_Nolineal) -> Transport Delay/1
  Sum8/1 -> ASIGNACION POLOS1/1
  PRIMERO ASIGNACION POLOS/1 -> Manual Switch/1
  Controlador FF3/1 -> Sum9/2
  Sum9/1 -> "MODELO SISTEMA CURVA REACCION "/1, Modelo_ Nolineal4/1(Q1)
  ASIGNACION POLOS1/1 -> Switch1/3
  Transport Delay/1 -> SALIDA (Cº)8/1
  Transport Delay1/1 -> SALIDA (Cº)9/2
  SALIDA (Cº)9/1 -> SALIDA (Cº)10/2
  SALIDA (Cº)10/1 -> Sum7/2, Sum8/2
  SALIDA (Cº)6/1 -> Scope5/1
  Sum7/1 -> CANCELACION POLOS1/1
  "MODELO SISTEMA CURVA REACCION "/1 -> SALIDA (Cº)11/1
  Constant7/1 -> SALIDA (Cº)11/2
  SALIDA (Cº)11/1 -> SALIDA (Cº)10/1, Transport Delay1/1
  PRIMERO CANCELACION POLOS/1 -> Manual Switch/2
  Manual Switch/1 -> Switch1/2
  PERTURBACION4/1 -> Controlador FF4/1, Modelo_ Nolineal5/2(Q2)
  PID Controller2/1 -> Scope6/2, Sum11/2
  REFERENCIA (Cº)2/1 -> Scope6/3
  Modelo_ Nolineal5/1(T1_Nolineal) -> SALIDA (Cº)13/1
  Band-Limited White Noise3/1 -> SALIDA (Cº)13/2
  SALIDA (Cº)12/1 -> Scope6/1
  SALIDA (Cº)13/1 -> Sum10/2, SALIDA (Cº)12/1
  Sum10/1 -> PID Controller2/1
  Controlador FF4/1 -> Sum11/1
  Transfer Fcn (with initial outputs)3/1 -> Sum10/1
  REFERENCIA5/1 -> Transfer Fcn (with initial outputs)3/1, REFERENCIA (Cº)2/1
  Sum11/1 -> Modelo_ Nolineal5/1(Q1)
  Constant8/1 -> SALIDA (Cº)12/2, REFERENCIA (Cº)2/2
  Constant9/1 -> SALIDA (Cº)14/2, REFERENCIA (Cº)3/2
  Controlador FF5/1 -> Sum13/1
  Sum12/1 -> PID Controller3/1
  REFERENCIA6/1 -> Transfer Fcn (with initial outputs)4/1, REFERENCIA (Cº)3/1
  Sum13/1 -> Modelo_ Nolineal6/1(Q1)
  SALIDA (Cº)14/1 -> Scope7/1
  Modelo_ Nolineal6/1(T1_Nolineal) -> SALIDA (Cº)14/1, Sum12/2
  PERTURBACION5/1 -> Controlador FF5/1, Modelo_ Nolineal6/2(Q2)
  PID Controller3/1 -> Scope7/2, Sum13/2
  Transfer Fcn (with initial outputs)4/1 -> Sum12/1
  REFERENCIA (Cº)3/1 -> Scope7/3

== system Modelo_benchmark/Modelo_ Nolineal ==
  Q1 : Inport
  Q2 : Inport  Port=2
  Subsystem : Subsystem
  T2_Nolineal : Subsystem
  T1_Nolineal : Outport
  T2_Nlineal : Outport  Port=2
  wires:
  Q2/1 -> T2_Nolineal/3(Q2)
  T2_Nolineal/1(T2_Nlineal) -> T2_Nlineal/1, Subsystem/2(T2_Nlineal), T2_Nolineal/2(T2_Nolineal)
  Subsystem/1(T1_Nolineal) -> T1_Nolineal/1, T2_Nolineal/1(T1_Nolineal)
  Q1/1 -> Subsystem/1(Q1)

== system Modelo_benchmark/Modelo_ Nolineal1 ==
  Q1 : Inport
  Q2 : Inport  Port=2
  Subsystem : Subsystem
  T2_Nolineal : Subsystem
  T1_Nolineal : Outport
  T2_Nlineal : Outport  Port=2
  wires:
  Q2/1 -> T2_Nolineal/3(Q2)
  T2_Nolineal/1(T2_Nlineal) -> T2_Nlineal/1, Subsystem/2(T2_Nlineal), T2_Nolineal/2(T2_Nolineal)
  Subsystem/1(T1_Nolineal) -> T1_Nolineal/1, T2_Nolineal/1(T1_Nolineal)
  Q1/1 -> Subsystem/1(Q1)

== system Modelo_benchmark/Modelo_ Nolineal2 ==
  Q1 : Inport
  Q2 : Inport  Port=2
  Subsystem : Subsystem
  T2_Nolineal : Subsystem
  T1_Nolineal : Outport
  T2_Nlineal : Outport  Port=2
  wires:
  Q2/1 -> T2_Nolineal/3(Q2)
  T2_Nolineal/1(T2_Nlineal) -> T2_Nlineal/1, Subsystem/2(T2_Nlineal), T2_Nolineal/2(T2_Nolineal)
  Subsystem/1(T1_Nolineal) -> T1_Nolineal/1, T2_Nolineal/1(T1_Nolineal)
  Q1/1 -> Subsystem/1(Q1)

== system Modelo_benchmark/Modelo_ Nolineal3 ==
  Q1 : Inport
  Q2 : Inport  Port=2
  Subsystem : Subsystem
  T2_Nolineal : Subsystem
  T1_Nolineal : Outport
  T2_Nlineal : Outport  Port=2
  wires:
  Q2/1 -> T2_Nolineal/3(Q2)
  T2_Nolineal/1(T2_Nlineal) -> T2_Nlineal/1, Subsystem/2(T2_Nlineal), T2_Nolineal/2(T2_Nolineal)
  Subsystem/1(T1_Nolineal) -> T1_Nolineal/1, T2_Nolineal/1(T1_Nolineal)
  Q1/1 -> Subsystem/1(Q1)

== system Modelo_benchmark/Modelo_ Nolineal4 ==
  Q1 : Inport
  Q2 : Inport  Port=2
  Subsystem : Subsystem
  T2_Nolineal : Subsystem
  T1_Nolineal : Outport
  T2_Nlineal : Outport  Port=2
  wires:
  Q2/1 -> T2_Nolineal/3(Q2)
  T2_Nolineal/1(T2_Nlineal) -> T2_Nlineal/1, Subsystem/2(T2_Nlineal), T2_Nolineal/2(T2_Nolineal)
  Subsystem/1(T1_Nolineal) -> T1_Nolineal/1, T2_Nolineal/1(T1_Nolineal)
  Q1/1 -> Subsystem/1(Q1)

== system Modelo_benchmark/Modelo_ Nolineal5 ==
  Q1 : Inport
  Q2 : Inport  Port=2
  Subsystem : Subsystem
  T2_Nolineal : Subsystem
  T1_Nolineal : Outport
  T2_Nlineal : Outport  Port=2
  wires:
  Q2/1 -> T2_Nolineal/3(Q2)
  T2_Nolineal/1(T2_Nlineal) -> T2_Nlineal/1, Subsystem/2(T2_Nlineal), T2_Nolineal/2(T2_Nolineal)
  Subsystem/1(T1_Nolineal) -> T1_Nolineal/1, T2_Nolineal/1(T1_Nolineal)
  Q1/1 -> Subsystem/1(Q1)

== system Modelo_benchmark/Modelo_ Nolineal6 ==
  Q1 : Inport
  Q2 : Inport  Port=2
  Subsystem : Subsystem
  T2_Nolineal : Subsystem
  T1_Nolineal : Outport
  T2_Nlineal : Outport  Port=2
  wires:
  Q2/1 -> T2_Nolineal/3(Q2)
  T2_Nolineal/1(T2_Nlineal) -> T2_Nlineal/1, Subsystem/2(T2_Nlineal), T2_Nolineal/2(T2_Nolineal)
  Subsystem/1(T1_Nolineal) -> T1_Nolineal/1, T2_Nolineal/1(T1_Nolineal)
  Q1/1 -> Subsystem/1(Q1)

== system Modelo_benchmark/Subsystem ==
  Q1 : Inport
  Q2 : Inport  Port=2
  Constant15 : Constant  Value=T1o
  Constant16 : Constant  Value=Tk
  GQ1T1 : TransferFcn  Numerator=[C1_Q1 C2_Q1]  Denominator=[P1_Q1 P2_Q1 P3_Q1]  ParameterTunability=Optimized
  GQ2T1 : TransferFcn  Numerator=[C1_Q2]  Denominator=[P1_Q2 P2_Q2 P3_Q2]  ParameterTunability=Optimized
  Q5 : Sum  Inputs=+++
  Step4 : Step  Time=300  After=13  SampleTime=0
  T1_lineal : Sum  Inputs=+-
  T1_nolineal1 : Sum  Inputs=+-
  T1_Lineal : Outport
  wires:
  T1_lineal/1 -> T1_Lineal/1
  T1_nolineal1/1 -> GQ1T1/1
  GQ1T1/1 -> Q5/1
  Constant16/1 -> T1_lineal/2
  Step4/1 -> T1_nolineal1/2
  GQ2T1/1 -> Q5/2
  Q5/1 -> T1_lineal/1
  Constant15/1 -> Q5/3
  Q2/1 -> GQ2T1/1
  Q1/1 -> T1_nolineal1/1

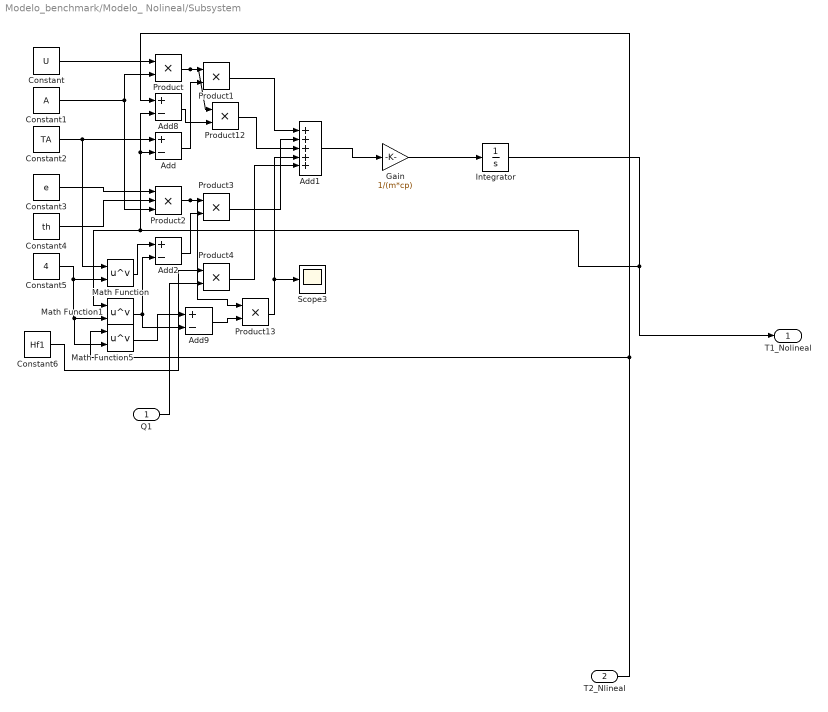
== system Modelo_benchmark/Modelo_ Nolineal/Subsystem ==
  Q1 : Inport
  T2_Nlineal : Inport  Port=2
  Add{,2,8..9} (4 alike) : Sum  Inputs=+-
  Add1 : Sum  Inputs=+++++
  Constant : Constant  Value=U
  Constant1 : Constant  Value=A
  Constant2 : Constant  Value=TA
  Constant3 : Constant  Value=e
  Constant4 : Constant  Value=th
  Constant5 : Constant  Value=4
  Constant6 : Constant  Value=Hf1
  Gain : Gain  Gain=1/(m*cp)
  Integrator : Integrator  InitialCondition=T1i
  Math Function : Math  Operator=pow
  Math Function1 : Math  Operator=pow
  Math Function5 : Math  Operator=pow
  Product{,1,3..4,12..13} (6 alike) : Product
  Product2 : Product  Inputs=3
  Scope3 : Scope
  T1_Nolineal : Outport
  wires:
  Add/1 -> Product1/2
  Constant4/1 -> Product2/2
  Math Function5/1 -> Add9/1
  T2_Nlineal/1 -> Math Function5/1, Add8/1
  Product/1 -> Product12/1, Product1/1
  Constant3/1 -> Product2/1
  Math Function1/1 -> Add2/2, Add9/2
  Constant6/1 -> Product4/1
  Product3/1 -> Add1/2
  Product13/1 -> Scope3/1, Add1/4
  Product12/1 -> Add1/3
  Constant5/1 -> Math Function5/2, Math Function1/2, Math Function/2
  Constant1/1 -> Product2/3, Product/2
  Product1/1 -> Add1/1
  Constant/1 -> Product/1
  Gain/1 -> Integrator/1
  Constant2/1 -> Math Function/1, Add/1
  Product4/1 -> Add1/5
  Integrator/1 -> T1_Nolineal/1, Math Function1/1, Add8/2, Add/2
  Add2/1 -> Product3/2
  Add1/1 -> Gain/1
  Q1/1 -> Product4/2
  Product2/1 -> Product13/1, Product3/1
  Add8/1 -> Product12/2
  Math Function/1 -> Add2/1
  Add9/1 -> Product13/2

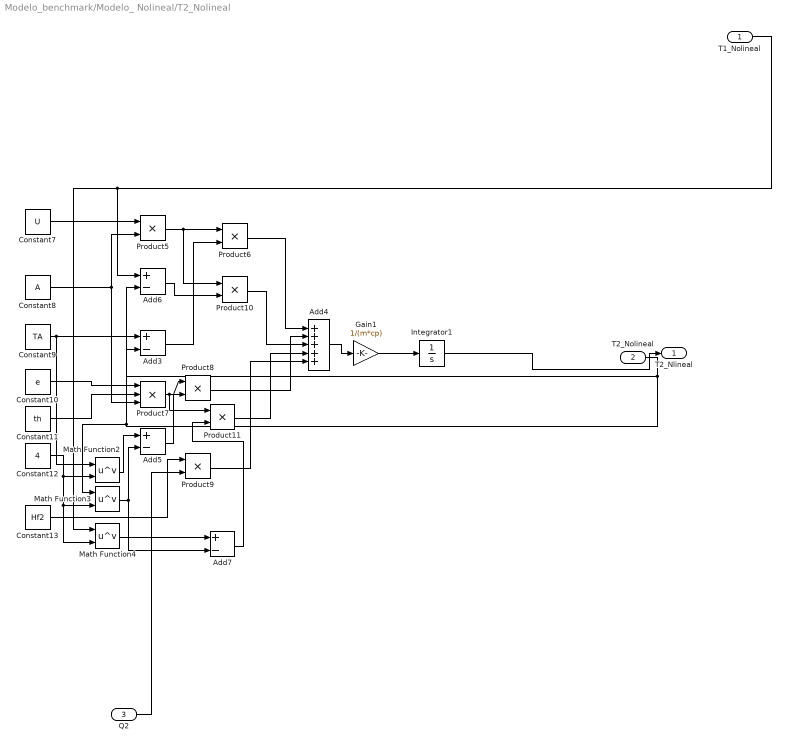
== system Modelo_benchmark/Modelo_ Nolineal/T2_Nolineal ==
  T1_Nolineal : Inport
  T2_Nolineal : Inport  Port=2
  Q2 : Inport  Port=3
  Add{3,5..7} (4 alike) : Sum  Inputs=+-
  Add4 : Sum  Inputs=+++++
  Constant10 : Constant  Value=e
  Constant11 : Constant  Value=th
  Constant12 : Constant  Value=4
  Constant13 : Constant  Value=Hf2
  Constant7 : Constant  Value=U
  Constant8 : Constant  Value=A
  Constant9 : Constant  Value=TA
  Gain1 : Gain  Gain=1/(m*cp)
  Integrator1 : Integrator  InitialCondition=T2i
  Math Function2 : Math  Operator=pow
  Math Function3 : Math  Operator=pow
  Math Function4 : Math  Operator=pow
  Product{5..6,8..11} (6 alike) : Product
  Product7 : Product  Inputs=3
  T2_Nlineal : Outport
  wires:
  Integrator1/1 -> T2_Nlineal/1
  Product11/1 -> Add4/4
  T2_Nolineal/1 -> Add3/2, Math Function3/1, Add6/2
  Product7/1 -> Product11/1, Product8/1
  Constant7/1 -> Product5/1
  Product8/1 -> Add4/2
  T1_Nolineal/1 -> Math Function4/1, Add6/1
  Product9/1 -> Add4/5
  Math Function3/1 -> Add7/2, Add5/2
  Add6/1 -> Product10/2
  Add3/1 -> Product6/2
  Constant9/1 -> Math Function2/1, Add3/1
  Constant12/1 -> Math Function4/2, Math Function3/2, Math Function2/2
  Add4/1 -> Gain1/1
  Add5/1 -> Product8/2
  Constant11/1 -> Product7/2
  Constant13/1 -> Product9/1
  Gain1/1 -> Integrator1/1
  Constant8/1 -> Product5/2, Product7/3
  Product10/1 -> Add4/3
  Math Function4/1 -> Add7/1
  Math Function2/1 -> Add5/1
  Product6/1 -> Add4/1
  Q2/1 -> Product9/2
  Constant10/1 -> Product7/1
  Product5/1 -> Product10/1, Product6/1
  Add7/1 -> Product11/2

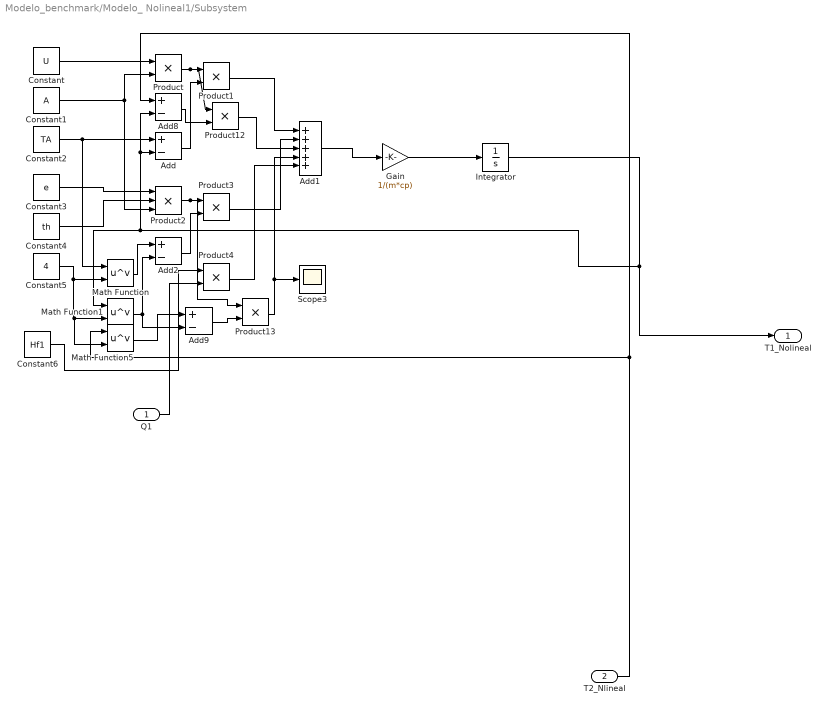
== system Modelo_benchmark/Modelo_ Nolineal1/Subsystem ==
  Q1 : Inport
  T2_Nlineal : Inport  Port=2
  Add{,2,8..9} (4 alike) : Sum  Inputs=+-
  Add1 : Sum  Inputs=+++++
  Constant : Constant  Value=U
  Constant1 : Constant  Value=A
  Constant2 : Constant  Value=TA
  Constant3 : Constant  Value=e
  Constant4 : Constant  Value=th
  Constant5 : Constant  Value=4
  Constant6 : Constant  Value=Hf1
  Gain : Gain  Gain=1/(m*cp)
  Integrator : Integrator  InitialCondition=T1i
  Math Function : Math  Operator=pow
  Math Function1 : Math  Operator=pow
  Math Function5 : Math  Operator=pow
  Product{,1,3..4,12..13} (6 alike) : Product
  Product2 : Product  Inputs=3
  Scope3 : Scope
  T1_Nolineal : Outport
  wires:
  Add/1 -> Product1/2
  Constant4/1 -> Product2/2
  Math Function5/1 -> Add9/1
  T2_Nlineal/1 -> Math Function5/1, Add8/1
  Product/1 -> Product12/1, Product1/1
  Constant3/1 -> Product2/1
  Math Function1/1 -> Add2/2, Add9/2
  Constant6/1 -> Product4/1
  Product3/1 -> Add1/2
  Product13/1 -> Scope3/1, Add1/4
  Product12/1 -> Add1/3
  Constant5/1 -> Math Function5/2, Math Function1/2, Math Function/2
  Constant1/1 -> Product2/3, Product/2
  Product1/1 -> Add1/1
  Constant/1 -> Product/1
  Gain/1 -> Integrator/1
  Constant2/1 -> Math Function/1, Add/1
  Product4/1 -> Add1/5
  Integrator/1 -> T1_Nolineal/1, Math Function1/1, Add8/2, Add/2
  Add2/1 -> Product3/2
  Add1/1 -> Gain/1
  Q1/1 -> Product4/2
  Product2/1 -> Product13/1, Product3/1
  Add8/1 -> Product12/2
  Math Function/1 -> Add2/1
  Add9/1 -> Product13/2

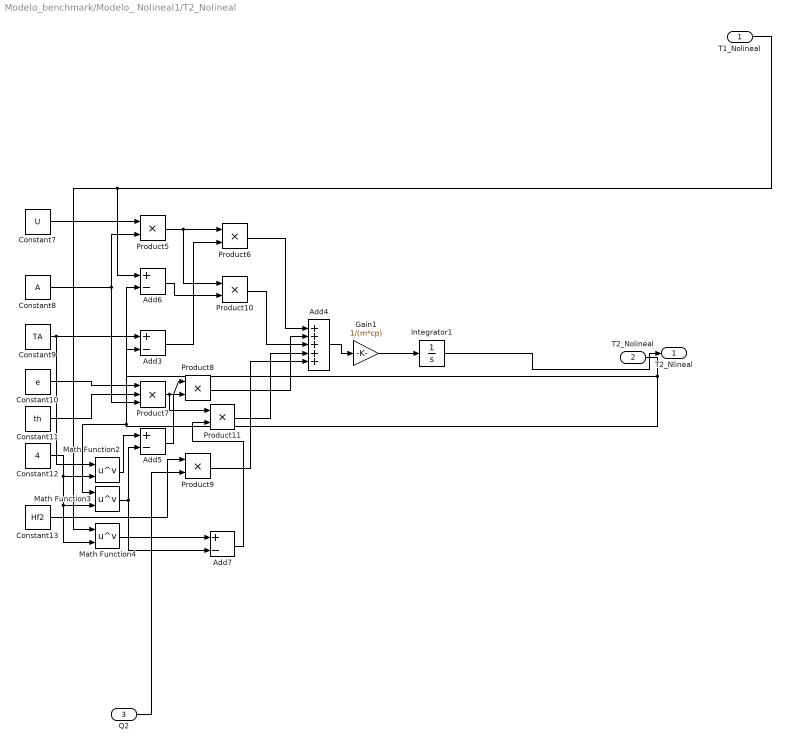
== system Modelo_benchmark/Modelo_ Nolineal1/T2_Nolineal ==
  T1_Nolineal : Inport
  T2_Nolineal : Inport  Port=2
  Q2 : Inport  Port=3
  Add{3,5..7} (4 alike) : Sum  Inputs=+-
  Add4 : Sum  Inputs=+++++
  Constant10 : Constant  Value=e
  Constant11 : Constant  Value=th
  Constant12 : Constant  Value=4
  Constant13 : Constant  Value=Hf2
  Constant7 : Constant  Value=U
  Constant8 : Constant  Value=A
  Constant9 : Constant  Value=TA
  Gain1 : Gain  Gain=1/(m*cp)
  Integrator1 : Integrator  InitialCondition=T2i
  Math Function2 : Math  Operator=pow
  Math Function3 : Math  Operator=pow
  Math Function4 : Math  Operator=pow
  Product{5..6,8..11} (6 alike) : Product
  Product7 : Product  Inputs=3
  T2_Nlineal : Outport
  wires:
  Integrator1/1 -> T2_Nlineal/1
  Product11/1 -> Add4/4
  T2_Nolineal/1 -> Add3/2, Math Function3/1, Add6/2
  Product7/1 -> Product11/1, Product8/1
  Constant7/1 -> Product5/1
  Product8/1 -> Add4/2
  T1_Nolineal/1 -> Math Function4/1, Add6/1
  Product9/1 -> Add4/5
  Math Function3/1 -> Add7/2, Add5/2
  Add6/1 -> Product10/2
  Add3/1 -> Product6/2
  Constant9/1 -> Math Function2/1, Add3/1
  Constant12/1 -> Math Function4/2, Math Function3/2, Math Function2/2
  Add4/1 -> Gain1/1
  Add5/1 -> Product8/2
  Constant11/1 -> Product7/2
  Constant13/1 -> Product9/1
  Gain1/1 -> Integrator1/1
  Constant8/1 -> Product5/2, Product7/3
  Product10/1 -> Add4/3
  Math Function4/1 -> Add7/1
  Math Function2/1 -> Add5/1
  Product6/1 -> Add4/1
  Q2/1 -> Product9/2
  Constant10/1 -> Product7/1
  Product5/1 -> Product10/1, Product6/1
  Add7/1 -> Product11/2

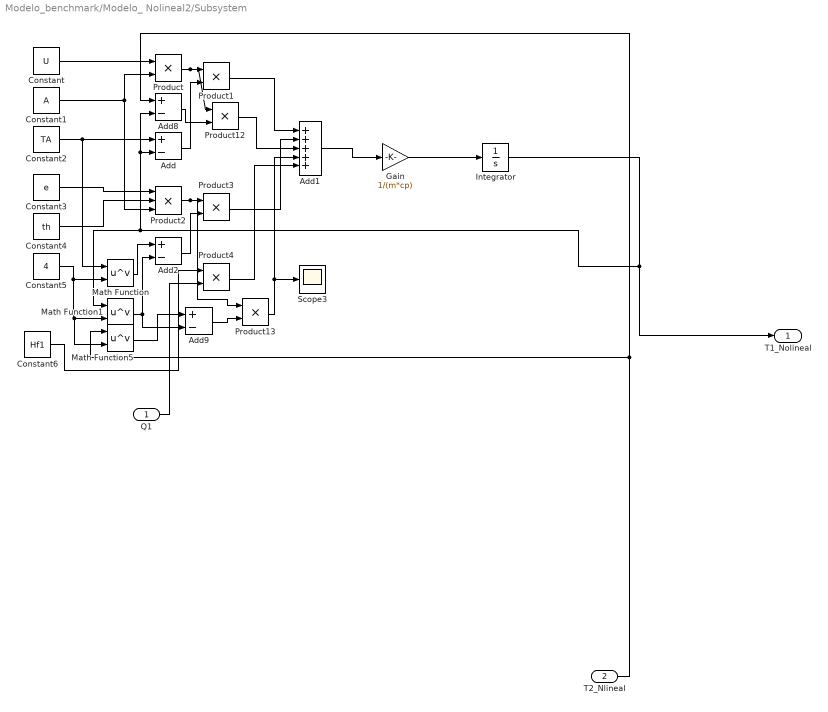
== system Modelo_benchmark/Modelo_ Nolineal2/Subsystem ==
  Q1 : Inport
  T2_Nlineal : Inport  Port=2
  Add{,2,8..9} (4 alike) : Sum  Inputs=+-
  Add1 : Sum  Inputs=+++++
  Constant : Constant  Value=U
  Constant1 : Constant  Value=A
  Constant2 : Constant  Value=TA
  Constant3 : Constant  Value=e
  Constant4 : Constant  Value=th
  Constant5 : Constant  Value=4
  Constant6 : Constant  Value=Hf1
  Gain : Gain  Gain=1/(m*cp)
  Integrator : Integrator  InitialCondition=T1i
  Math Function : Math  Operator=pow
  Math Function1 : Math  Operator=pow
  Math Function5 : Math  Operator=pow
  Product{,1,3..4,12..13} (6 alike) : Product
  Product2 : Product  Inputs=3
  Scope3 : Scope
  T1_Nolineal : Outport
  wires:
  Add/1 -> Product1/2
  Constant4/1 -> Product2/2
  Math Function5/1 -> Add9/1
  T2_Nlineal/1 -> Math Function5/1, Add8/1
  Product/1 -> Product12/1, Product1/1
  Constant3/1 -> Product2/1
  Math Function1/1 -> Add2/2, Add9/2
  Constant6/1 -> Product4/1
  Product3/1 -> Add1/2
  Product13/1 -> Scope3/1, Add1/4
  Product12/1 -> Add1/3
  Constant5/1 -> Math Function5/2, Math Function1/2, Math Function/2
  Constant1/1 -> Product2/3, Product/2
  Product1/1 -> Add1/1
  Constant/1 -> Product/1
  Gain/1 -> Integrator/1
  Constant2/1 -> Math Function/1, Add/1
  Product4/1 -> Add1/5
  Integrator/1 -> T1_Nolineal/1, Math Function1/1, Add8/2, Add/2
  Add2/1 -> Product3/2
  Add1/1 -> Gain/1
  Q1/1 -> Product4/2
  Product2/1 -> Product13/1, Product3/1
  Add8/1 -> Product12/2
  Math Function/1 -> Add2/1
  Add9/1 -> Product13/2
